simulink model "signal_detector_V2"  (R2018a)
settings: Solver=VariableStepAuto  StartTime=0.0  StopTime=inf  RelTol=1e-3
StartFcn:
  | localAddEventListener
undefined symbols (not defined in the file or in its folder): magnitude
libraries: dspstat3 x3, dsparch4 x2, dspmlti4 x2, rtlsdr_book_library x1, dspsnks4 x1, sdrrlib x1, commrflib2 x1
settings Model: Creator=amitm  LastModifiedBy=amitm
settings OptimizationCC: BlockReduction=off

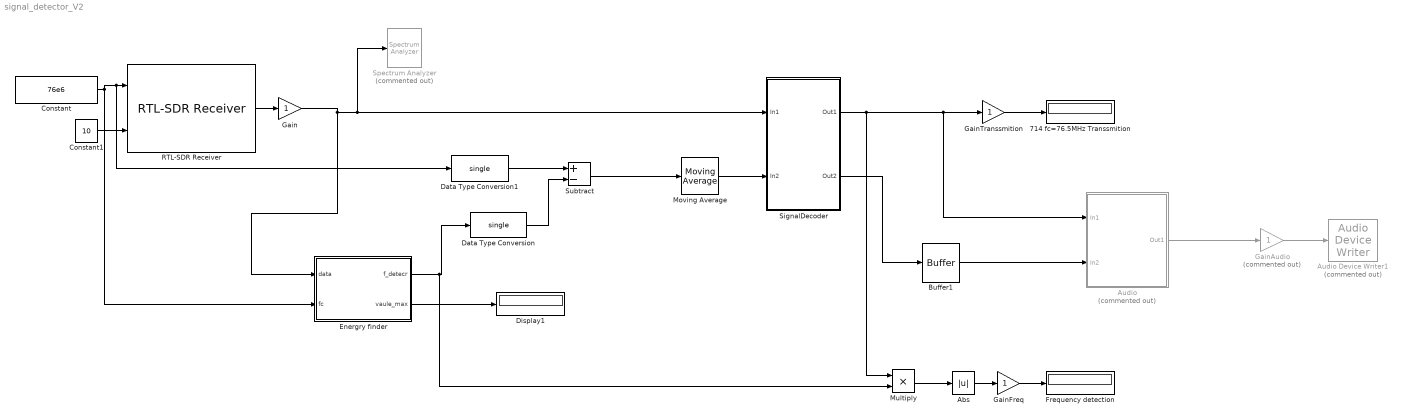
== system signal_detector_V2 ==
  714 fc=76.5MHz Transsmition : Display
  Abs : Abs
  "Audio " : Subsystem  Commented=on
  Audio Device Writer1 : dspsnks4/Audio Device Writer  Commented=on  Driver=DirectSound  Device=Speakers (Realtek(R) Audio)  InheritSampleRate=off  SampleRate=48e3  BitDepth=16-bit integer  BufferSize=4096  NumBuffers=10  DefaultOutputChannelMapping=on  OutputChannelMapping=1:2  OutputNumUnderrunSamples=off  DriverIdx=1  DeviceWarnFlag=''
  Buffer1 : Buffer  N=80  OutputFrames=off
  Constant : Constant  Value=76e6
  Constant1 : Constant  Value=10
  Data Type Conversion : DataTypeConversion  OutDataTypeStr=single
  Data Type Conversion1 : DataTypeConversion  OutDataTypeStr=single
  Display1 : Display
  Energry finder : MATLAB Function  TreatAsAtomicUnit=on
  Frequency detection : Display
  Gain : Gain
  GainAudio : Gain  Commented=on
  GainFreq : Gain
  GainTranssmition : Gain
  Moving Average : dspstat3/Moving Average  Method=Sliding window  ForgettingFactorPort=off  SpecifyWindowLength=on  WindowLength=16  ForgettingFactor=0.9  SimulateUsing=Code generation
  Multiply : Product
  RTL-SDR Receiver : sdrrlib/RTL-SDR Receiver  IPAddress=0  CenterFrequencySource=Input port  CenterFrequency=102.5e6  GainSource=Input port  Gain=0  ADCRate=2.4e6  FrequencyCorrection=0  LostSamplesOutputPort=off  LatencyOutputPort=off  OutputDataType=single  FrameLength=2^12  EnableBurstMode=off  NumFramesInBurst=20  sobjType=sdrr.internal.SDRRTLReceiverSL  dataUDPPort=-1  ctrlUDPPort=-1  subDeviceList=nosubdev  sdrBlockType=SDRBlockTypeSLT.SDRRxBlock  requester=UNUSED_BY_SFCN  sdrExecutionMode=SDRExecutionModeSLT.ExecModeHW  BypassUserLogic=off  DecimatorSelect=DDC decimator  SourceSelect=RF data  SineAmplitude=16000  EnableInternalClock=off  BypassIQBalance=off  IFBandwidth=40e6  ADCRateSource=Dialog  IntermediateFrequency=0  DecimationFactorSource=Dialog  DecimationFactor=512  RFFrequencyIsTunable=logical(1)  SampleTime=(2^12)/(2.4e6)  IFBandwidthSource=Dialog  SineFrequency=30000  BypassDCBlockingFilter=off  IntermediateFrequencySource=Dialog  IQBalanceCoefficients=64  SkipAllHardwareResetAndInitialization=off  EnableIQCalibrationTable=on  CacheIQCalibrationTable=off  EnableOffsetTuning=off  EnableRTLAGC=off  EnableTestMode=off  EnableTunerAGC=on  FrequencyCorrectionSource=Dialog  NumMLBuffers=128  NumUSBBuffers=16  RTLCrystalFrequency=28800000  TunerCrystalFrequency=28800000
      settings: SourceProductName=Communications System Toolbox Support Package for RTL-SDR Radio  SourceProductBaseCode=RTLSDR
  SignalDecoder : Subsystem
  Spectrum Analyzer : SpectrumAnalyzer  Commented=on
  Subtract : Sum  Inputs=+-
  wires:
  Moving Average/1 -> SignalDecoder/2(In2)
  Constant/1 -> Data Type Conversion1/1, RTL-SDR Receiver/1, Energry finder/2(fc)
  Subtract/1 -> Moving Average/1
  Data Type Conversion1/1 -> Subtract/1
  Energry finder/2(vaule_max) -> Display1/1
  Constant1/1 -> RTL-SDR Receiver/2
  Energry finder/1(f_detecr) -> Multiply/2, Data Type Conversion/1
  Data Type Conversion/1 -> Subtract/2
  RTL-SDR Receiver/1 -> Gain/1
  Buffer1/1 -> "Audio "/2(In2)
  SignalDecoder/1(Out1) -> Multiply/1, GainTranssmition/1, "Audio "/1(In1)
  SignalDecoder/2(Out2) -> Buffer1/1
  Multiply/1 -> Abs/1
  Abs/1 -> GainFreq/1
  Gain/1 -> Spectrum Analyzer/1, SignalDecoder/1(In1), Energry finder/1(data)
  GainTranssmition/1 -> 714 fc=76.5MHz Transsmition/1
  GainFreq/1 -> Frequency detection/1
  GainAudio/1 -> Audio Device Writer1/1
  "Audio "/1(Out1) -> GainAudio/1

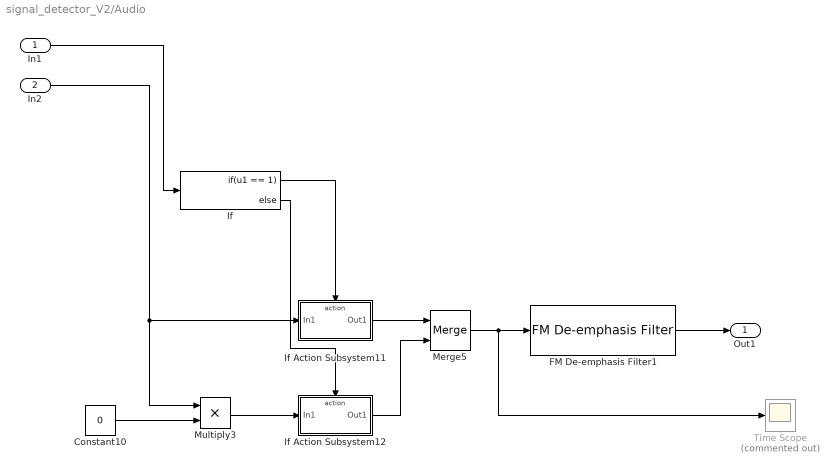
== system signal_detector_V2/Audio  ==
  In1 : Inport
  In2 : Inport  Port=2
  Constant10 : Constant  Value=0  OutDataTypeStr=single
  FM De-emphasis Filter1 : rtlsdr_book_library/FM Demod Tools/FM De-emphasis Filter  region=Europe, Asia  fs=48e3
      settings: SourceProductName=RTL-SDR Book Library
  If : If  IfExpression=u1 == 1
  If Action Subsystem11 : Subsystem  TreatAsAtomicUnit=on
  If Action Subsystem12 : Subsystem  TreatAsAtomicUnit=on
  Merge5 : Merge
  Multiply3 : Product
  Time Scope : Scope  Commented=on
  Out1 : Outport
  wires:
  In1/1 -> If/1
  Merge5/1 -> Time Scope/1, FM De-emphasis Filter1/1
  Multiply3/1 -> If Action Subsystem12/1(In1)
  If Action Subsystem12/1(Out1) -> Merge5/2
  If/2 -> If Action Subsystem12/Action
  If Action Subsystem11/1(Out1) -> Merge5/1
  Constant10/1 -> Multiply3/2
  If/1 -> If Action Subsystem11/Action
  FM De-emphasis Filter1/1 -> Out1/1
  In2/1 -> Multiply3/1, If Action Subsystem11/1(In1)

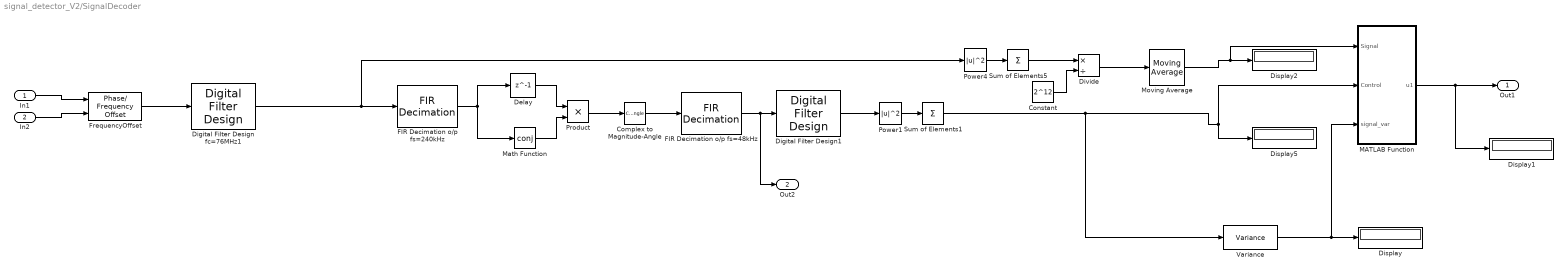
== system signal_detector_V2/SignalDecoder ==
  In1 : Inport
  In2 : Inport  Port=2
  Complex to Magnitude-Angle : ComplexToMagnitudeAngle  Output=Angle
  Constant : Constant  Value=2^12
  Delay : Delay  DelayLength=1  InputProcessing=Columns as channels (frame based)
  Digital Filter Design fc=76MHz1 : dsparch4/Digital Filter Design  mwdsp_browser_bugfix_var=off
  Digital Filter Design1 : dsparch4/Digital Filter Design  mwdsp_browser_bugfix_var=off
  Display{,1..2,5} (4 alike) : Display
  Divide : Product  Inputs=*/
  FIR Decimation o/p fs=240kHz : dspmlti4/FIR Decimation  FilterSource=Dialog parameters  h=firpm(50,[0 120e3 240e3 (2.4e6/2)]/(2.4e6/2),[1 1 0 0],[1 1],20)  D=10  filtStruct=Direct form  FilterObject=FDECIM  InputProcessing=Columns as channels (frame based)  framing=Allow multirate processing  inputOffset=0  outputBufInitCond=0  roundingMode=Floor  overflowMode=off  firstCoeffDataTypeStr=Inherit: Same word length as input  firstCoeffMin=[]  firstCoeffMax=[]  firstCoeffLastDataTypeStr=Inherit: Same word length as input  outputDataTypeStr=Inherit: Same as accumulator  outputMin=[]  outputMax=[]  outputLastDataTypeStr=Inherit: Same as accumulator
  FIR Decimation o/p fs=48kHz : dspmlti4/FIR Decimation  FilterSource=Dialog parameters  h=firpm(50,[0 15e3 20e3 (240e3/2)]/(240e3/2),[1 1 0 0],[1 1],20)  D=5  filtStruct=Direct form  FilterObject=FDECIM  InputProcessing=Columns as channels (frame based)  framing=Allow multirate processing  inputOffset=0  outputBufInitCond=0  roundingMode=Floor  overflowMode=off  firstCoeffDataTypeStr=Inherit: Same word length as input  firstCoeffMin=[]  firstCoeffMax=[]  firstCoeffLastDataTypeStr=Inherit: Same word length as input  outputDataTypeStr=Inherit: Same as accumulator  outputMin=[]  outputMax=[]  outputLastDataTypeStr=Inherit: Same as accumulator
  FrequencyOffset : commrflib2/Phase// Frequency Offset  phaseOffset=0  freqPort=on  freqOffset=-0.5e6
      settings: SourceProductName=Communications System Toolbox
  MATLAB Function : MATLAB Function  TreatAsAtomicUnit=on
  Math Function : Math  Operator=conj  SaturateOnIntegerOverflow=on
  Moving Average : dspstat3/Moving Average  Method=Sliding window  ForgettingFactorPort=off  SpecifyWindowLength=on  WindowLength=8  ForgettingFactor=0.9  SimulateUsing=Code generation
  Power1 : Math  Operator=magnitude^2  SaturateOnIntegerOverflow=on
  Power4 : Math  Operator=magnitude^2  SaturateOnIntegerOverflow=on
  Product : Product
  Sum of Elements1 : Sum  Inputs=+
  Sum of Elements5 : Sum  Inputs=+
  Variance : dspstat3/Variance  run=on  InputProcessing=Columns as channels (frame based)  reset_popup=None  directionMode=Each column  dimension=1  roiEnable=off  roiType=Rectangles  roiPortion=Entire ROI  roiOutput=Individual statistics for each ROI  roiFlag=off  roundingMode=Floor  overflowMode=off
      settings: SourceProductName=DSP System Toolbox
  Out1 : Outport
  Out2 : Outport  Port=2
  wires:
  FrequencyOffset/1 -> Digital Filter Design fc=76MHz1/1
  Power1/1 -> Sum of Elements1/1
  FIR Decimation o/p fs=48kHz/1 -> Out2/1, Digital Filter Design1/1
  Sum of Elements1/1 -> Variance/1, Display5/1, MATLAB Function/2(Control)
  Digital Filter Design1/1 -> Power1/1
  Complex to Magnitude-Angle/1 -> FIR Decimation o/p fs=48kHz/1
  FIR Decimation o/p fs=240kHz/1 -> Math Function/1, Delay/1
  Product/1 -> Complex to Magnitude-Angle/1
  Digital Filter Design fc=76MHz1/1 -> Power4/1, FIR Decimation o/p fs=240kHz/1
  Power4/1 -> Sum of Elements5/1
  Delay/1 -> Product/1
  Math Function/1 -> Product/2
  Variance/1 -> MATLAB Function/3(signal_var), Display/1
  In1/1 -> FrequencyOffset/1
  In2/1 -> FrequencyOffset/2
  MATLAB Function/1(u1) -> Display1/1, Out1/1
  Sum of Elements5/1 -> Divide/1
  Constant/1 -> Divide/2
  Divide/1 -> Moving Average/1
  Moving Average/1 -> MATLAB Function/1(Signal), Display2/1

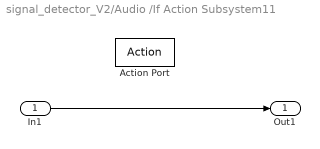
== system signal_detector_V2/Audio /If Action Subsystem11 ==
  In1 : Inport
  Action Port : ActionPort  ActionType=then
  Out1 : Outport
  wires:
  In1/1 -> Out1/1

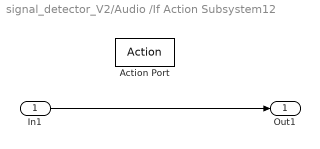
== system signal_detector_V2/Audio /If Action Subsystem12 ==
  In1 : Inport
  Action Port : ActionPort  ActionType=else
  Out1 : Outport
  wires:
  In1/1 -> Out1/1

== matlab function signal_detector_V2/Energry finder ==
  data: data input; f_detecr output; vaule_max output; fc input
function [f_detecr,vaule_max] = fcn(data,fc)


% fc = 76e6;
fs = 2.4e6;
data_points = 2^12;

% signal = data.Data(10,:);
signal = data;
freq = linspace(-fs/2+fc,fs/2+fc,data_points);
power = (fftshift(fft(signal))/length(signal));


[vaule_max,index_max] = max(abs(power));
f_detecr = freq(index_max);

== matlab function signal_detector_V2/SignalDecoder/MATLAB Function ==
  data: Signal input; u1 output; Control input; signal_var input
function u1   = fcn(Signal,Control,signal_var)

threshold_signal = 0.03;
threshold_control = 0.1;
threshold_signal_var = 150;



if Signal > threshold_signal && Control>threshold_control 
    u1 = 1;
elseif Signal > threshold_signal 
    u1=-1;
else
    u1 = 0;
end
